simulink model "slo_single_share"  (R2015b)
settings: Solver=FixedStepDiscrete  SolverMode=SingleTasking  StartTime=0.0  StopTime=10  RelTol=1e-3
libraries: dspsrcs4 x1
settings Model: DataTypeOverride=Off  Creator=amatsumo  LastModifiedBy=amatsumo
settings DataIOCC: SaveFormat=Array  SaveOutput=off  SignalLogging=off  SaveTime=off
settings OptimizationCC: BlockReduction=off  ConditionallyExecuteInputs=off  DefaultParameterBehavior=Inlined
settings DebuggingCC: AlgebraicLoopMsg=error  UnderspecifiedInitializationDetection=Classic  MergeDetectMultiDrivingBlocksExec=none  SolverPrmCheckMsg=warning  SingleTaskRateTransMsg=error  StateNameClashWarn=warning
settings HardwareCC: ProdBitPerPointer=32  ProdLargestAtomicFloat=None  ProdIntDivRoundTo=Undefined  ProdEndianess=Unspecified  ProdWordSize=32  ProdHWDeviceType=ASIC/FPGA->ASIC/FPGA  ProdEqTarget=off
settings GRTTargetCC: GeneratePreprocessorConditionals=Disable all
settings ConfigComp: CovModelRefEnable=Off  CovSFcnEnable=off

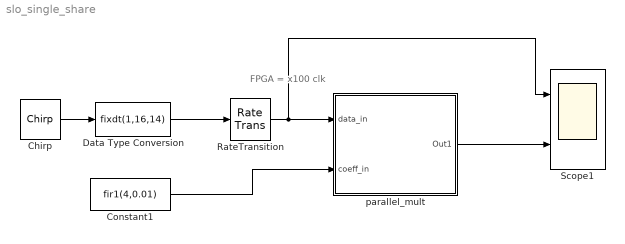
== system slo_single_share ==
  note: FPGA =
      | x100 clk
  Chirp : dspsrcs4/Chirp  sweep=Linear  mode=Unidirectional  f0=10  f1=50e3  t1=10  Tsweep=10  phase=0  Ts=1/100e3  spf=1  datatype=Double  OutputFrames=on
  Constant1 : Constant  Value=fir1(4,0.01)  OutDataTypeStr=fixdt(1,16,14)  SampleTime=-1
  Data Type Conversion : DataTypeConversion  OutDataTypeStr=fixdt(1,16,14)
  RateTransition : RateTransition  OutPortSampleTimeOpt=Multiple of input port sample time  OutPortSampleTimeMultiple=1 %1/100  OutPortSampleTime=2e-6
  Scope1 : Scope  NumInputPorts=2
  parallel_mult : Subsystem
  wires:
  Chirp/1 -> Data Type Conversion/1
  Data Type Conversion/1 -> RateTransition/1
  Constant1/1 -> parallel_mult/2(coeff_in)
  parallel_mult/1(Out1) -> Scope1/2
  RateTransition/1 -> Scope1/1, parallel_mult/1(data_in)

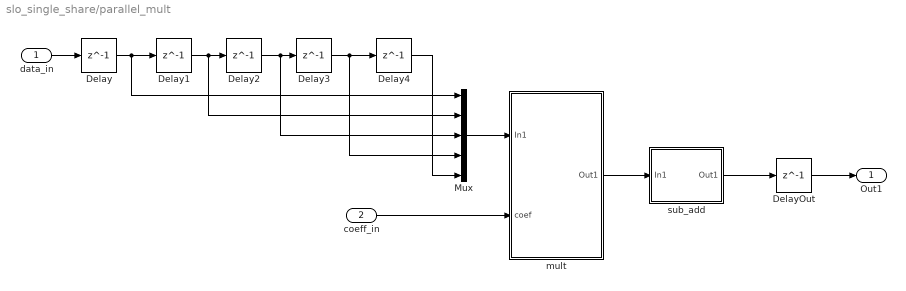
== system slo_single_share/parallel_mult ==
  data_in : Inport
  coeff_in : Inport  Port=2
  Delay{,1..4} (5 alike) : Delay  DelayLength=1
  DelayOut : Delay  DelayLength=1
  Mux : Mux  Inputs=5
  mult : Subsystem
  sub_add : Subsystem
  Out1 : Outport
  wires:
  mult/1(Out1) -> sub_add/1(In1)
  data_in/1 -> Delay/1
  coeff_in/1 -> mult/2(coef)
  Delay/1 -> Mux/1, Delay1/1
  Delay2/1 -> Mux/3, Delay3/1
  Delay3/1 -> Mux/4, Delay4/1
  Delay1/1 -> Mux/2, Delay2/1
  sub_add/1(Out1) -> DelayOut/1
  Delay4/1 -> Mux/5
  Mux/1 -> mult/1(In1)
  DelayOut/1 -> Out1/1

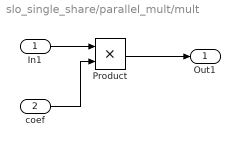
== system slo_single_share/parallel_mult/mult ==
  In1 : Inport
  coef : Inport  Port=2
  Product : Product  RndMeth=Zero
  Out1 : Outport
  wires:
  In1/1 -> Product/1
  Product/1 -> Out1/1
  coef/1 -> Product/2

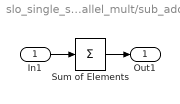
== system slo_single_share/parallel_mult/sub_add ==
  In1 : Inport
  Sum of Elements : Sum  Inputs=+
  Out1 : Outport
  wires:
  Sum of Elements/1 -> Out1/1
  In1/1 -> Sum of Elements/1
